simulink model "SCRReferenceApplication"  (R2021a)
settings: Solver=ode23tb  StartTime=0.0  StopTime=20  RelTol=2e-1
model workspace (MAT data in the model file):
  EngPwr = 352122.842504
  EngWc = 4.047
  Tdiff = 849
  Tlim = 1000
  VEH.Mass = 1181
  VEH.StaticNormalFrontLoad.FR = 264.666666667
  VEH.StaticNormalFrontLoad.FL = 264.666666667
  VEH.StaticNormalRearLoad.RR = 322
  VEH.StaticNormalRearLoad.RL = 322
  VEH.WheelBase = 3.075
  VEH.FrontAxlePositionfromCG = 1.515
  VEH.RearAxlePositionfromCG = 1.504
  VEH.HeightCG = 0.134
  VEH.FrontalArea = 2.11
  VEH.DragCoefficient = 0.33
  VEH.NumberOfWheelsPerAxle = 2
  VEH.Thread.FR = 1.705
  VEH.Thread.RR = 1.705
  VEH.PitchMomentInertia = 1922.66666667
  VEH.RollMomentInertia = 432.333333333
  VEH.YawMomentInertia = 2066
  VEH.SteeringRatio = 18
  VEH.TrackWidth = 1.922
  VEH.SprungMass = 1096.72266667
  VEH.InitialLongPosition = 0
  VEH.InitialLatPosition = 3.125
  VEH.InitialVertPosition = 0.0111
  VEH.InitialRollAngle = 0
  VEH.InitialPitchAngle = -0.000732
  VEH.InitialYawAngle = 0
  VEH.InitialLongVel = 0
  VEH.InitialLatVel = 0
  VEH.InitialVertVel = 0
  VEH.InitialRollRate = 0
  VEH.InitialPitchRate = 0
  VEH.InitialYawRate = 0
libraries: sim3dlib x3, Solver_SF x1, vdynlib x1, simulink x1
settings Model: ModifiedByFormat=The MathWorks, Inc.  SimulationMode=accelerator  Creator=The MathWorks, Inc.  LastModifiedBy=The MathWorks, Inc.
settings SolverCC: SolverJacobianMethodControl=FullPerturbation  ZeroCrossAlgorithm=Adaptive  AlgebraicLoopSolver=TrustRegion  DecoupledContinuousIntegration=on  MinimalZcImpactIntegration=on
settings DataIOCC: ReturnWorkspaceOutputs=off  Refine=2
settings DebuggingCC: IgnoredZcDiagnostic=none  PregeneratedLibrarySubsystemCodeDiagnostic=none  SFMachineParentedDataDiag=warning  ArithmeticOperatorsInVariantConditions=warning
settings ModelReferenceCC: ModelReferenceMinAlgLoopOccurrences=on
settings SFSimCC: SimUseLocalCustomCode=off
settings RTWCC: RTWUseLocalCustomCode=off

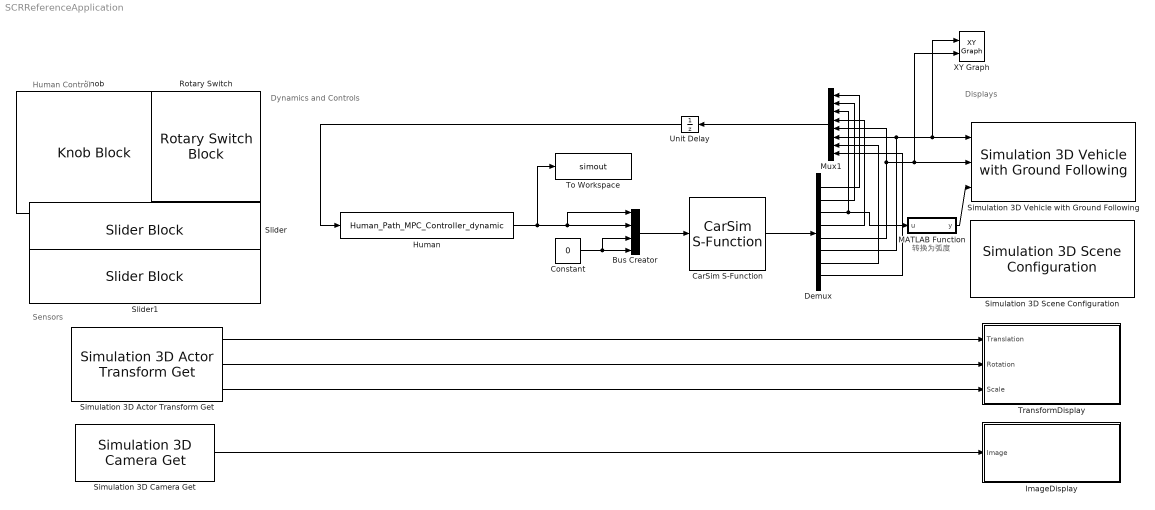
== system SCRReferenceApplication ==
  note: 转换为弧度
  note: Displays
  note: Dynamics and Controls
  note: Sensors
  note: Human Control
  Bus Creator : BusCreator  Inputs=4
  CarSim S-Function : Solver_SF/CarSim S-Function  Priority=1  SIMFILE=simfile.sim  Run_RTs=off  vs_state_ind=Run  StopMode_ind=Vehicle Model
  Constant : Constant  Value=0
  Demux : Demux  Outputs=8
  Human : S-Function  FunctionName=Human_Path_MPC_Controller_dynamic  SFunctionDeploymentMode=off  EnableBusSupport=off
  ImageDisplay : Subsystem
  Knob : KnobBlock  LabelPosition=Bottom  ScaleMin=-90  ScaleMax=90  TickInterval=30
  MATLAB Function : MATLAB Function  TreatAsAtomicUnit=on
  Mux1 : Mux  Inputs=8
  Rotary Switch : RotarySwitchBlock  LabelPosition=Bottom
      settings: Values={{'R', 'N', 'D'}, [-1 0 1]}
  Simulation 3D Actor Transform Get : sim3dlib/Simulation 3D Actor Transform Get  Priority=1  ActorTag=SimulinkVehicle1  NumberOfParts=5  CustNumOfParts=3  Ts=-1  aMode=2
      settings: SourceProductBaseCode=DR,UV,VE
  Simulation 3D Camera Get : sim3dlib/Simulation 3D Camera Get  Priority=1  sensorTag=Sim3dSensor1  sensorId=1  sensorName=Sim3dSensor1  vehTagList={'Scene Origin';'SimulinkVehicle1'}  vehTag=SimulinkVehicle1  mountLoc=Rearview mirror  offsetFlag=off  tmountOffset=[0, 0, 0]  rmountOffset=[0, 0, 0]  HorizontalResolution=1024  VerticalResolution=768  HorizontalFOV=90  SampleTime=.03  mountPoint=[0.319999992847443 0 1.19000005722046]  mountOrientation=[0 0 0]  aMode=2  ID=1
      settings: SourceProductBaseCode=DR,UV,VE
  Simulation 3D Scene Configuration : sim3dlib/Simulation 3D Scene Configuration  Priority=0  ProjectFormat=Default Scenes  SceneDesc=Straight road  ProjectName=F:\MATLAB\R2021a\toolbox\shared\sim3d_projects\automotive_project\UE4\WindowsNoEditor\VehicleSimulation.exe  ScenePath=/Game/Maps/HwStrght  vehTagList={'Scene Origin';'SimulinkVehicle1'}  vehTag=SimulinkVehicle1  OpVisEn=off  Ts=.03  EnableWindow=on  EnableWeather=off  SunAltitude=60  SunAzimuth=90  clouds=40  wind=1  fog=0  rain=0  sensorTag=MainCamera1  sensorId=1  sensorName=MainCamera1  mountLoc=Origin  offsetFlag=off  tmountOffset=[0, 0, 0]  rmountOffset=[0, 0, 0]  HorizontalResolution=1280  VerticalResolution=720  HorizontalFOV=60  mountPoint=[0 0 0]  mountOrientation=[0 0 0]  aMode=2  ID=1
      settings: SourceProductBaseCode=DR,UV,VE
  Simulation 3D Vehicle with Ground Following : vdynlib/Vehicle Scenarios/Sim3D/Sim3D Vehicle/Components/Simulation 3D Vehicle with Ground Following  Priority=-1  PassVehMesh=Muscle car  MeshPath=/MathWorksSimulation/Vehicles/Muscle/Meshes/SK_MuscleCar.SK_MuscleCar  TrackWidth=1.9  WheelBase=3  WheelRadius=0.35  VehColor=Red  InitialPos=[0, 0, 0]  InitialRot=[0, 0, 0]  ActorName=SimulinkVehicle1  VehLightsControl=off  HeadlightColor=[ 1, 1, 1 ]  HighBeamIntensity=100000  LowBeamIntensity=60000  HighBeamConeAngle=1.22  LowBeamConeAngle=1.22  LeftHeadlightOrientation=[ 0, 0 ]  RightHeadlightOrientation=[ 0, 0 ]  BrakelightIntensity=200  ReverselightIntensity=500  SignallightIntensity=500  SignallightPeriod=1  SignalPulseWidth=50  SampleTime=-1  ActorType=SimulinkVehicle  ID=1  aMode=2  ActorTag=SimulinkVehicle1  CoordinateScheme=SAE
      settings: SourceProductBaseCode=VE
  Slider : SliderBlock  LabelPosition=Bottom  ScaleMax=1  TickInterval=.2
  Slider1 : SliderBlock  LabelPosition=Bottom  ScaleMax=1  TickInterval=.2
  To Workspace : ToWorkspace  VariableName=simout  SaveFormat=Timeseries  SampleTime=-1
  TransformDisplay : Subsystem
  Unit Delay : UnitDelay  SampleTime=-1  HasFrameUpgradeWarning=on
  XY Graph : simulink/Sinks/XY Graph  xmin=-5  xmax=200  ymin=-2  ymax=10  st=-1
  wires:
  Simulation 3D Camera Get/1 -> ImageDisplay/1(Image)
  Simulation 3D Actor Transform Get/1 -> TransformDisplay/1(Translation)
  Simulation 3D Actor Transform Get/2 -> TransformDisplay/2(Rotation)
  Simulation 3D Actor Transform Get/3 -> TransformDisplay/3(Scale)
  CarSim S-Function/1 -> Demux/1
  Mux1/1 -> Unit Delay/1
  Unit Delay/1 -> Human/1
  MATLAB Function/1(y) -> Simulation 3D Vehicle with Ground Following/3
  Demux/2 -> Mux1/2
  Demux/3 -> MATLAB Function/1(u), Mux1/3
  Demux/4 -> Mux1/4
  Demux/5 -> XY Graph/2, Simulation 3D Vehicle with Ground Following/2, Mux1/5
  Demux/6 -> XY Graph/1, Simulation 3D Vehicle with Ground Following/1, Mux1/6
  Demux/1 -> Mux1/1
  Demux/7 -> Mux1/7
  Demux/8 -> Mux1/8
  Constant/1 -> Bus Creator/3, Bus Creator/4
  Bus Creator/1 -> CarSim S-Function/1
  Human/1 -> To Workspace/1, Bus Creator/1, Bus Creator/2

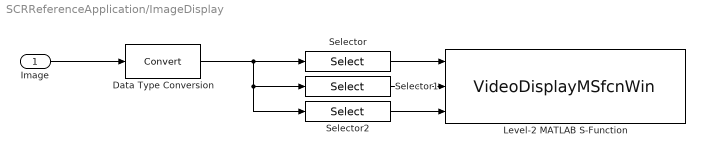
== system SCRReferenceApplication/ImageDisplay ==
  Image : Inport
  Data Type Conversion : DataTypeConversion
  Level-2 MATLAB S-Function : M-S-Function  FunctionName=VideoDisplayMSfcnWin  Parameters=1
  Selector : Selector  NumberOfDimensions=3  InputPortWidth=3  IndexOptions=Select all,Select all,Index vector (dialog)  Indices=[1 3],1,1  OutputSizes=1,1,1
  Selector1 : Selector  NumberOfDimensions=3  InputPortWidth=3  IndexOptions=Select all,Select all,Index vector (dialog)  Indices=[1 3],1,2  OutputSizes=1,1,1
  Selector2 : Selector  NumberOfDimensions=3  InputPortWidth=3  IndexOptions=Select all,Select all,Index vector (dialog)  Indices=[1 3],1,3  OutputSizes=1,1,1
  wires:
  Data Type Conversion/1 -> Selector2/1, Selector1/1, Selector/1
  Image/1 -> Data Type Conversion/1
  Selector1/1 -> Level-2 MATLAB S-Function/2
  Selector2/1 -> Level-2 MATLAB S-Function/3
  Selector/1 -> Level-2 MATLAB S-Function/1

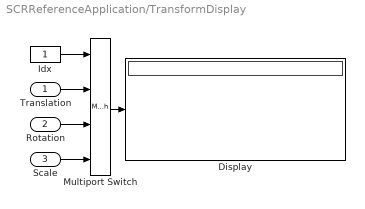
== system SCRReferenceApplication/TransformDisplay ==
  Translation : Inport
  Rotation : Inport  Port=2
  Scale : Inport  Port=3
  " Multiport Switch" : MultiPortSwitch
  Display : Display
  Idx : Constant
  wires:
  " Multiport Switch"/1 -> Display/1
  Idx/1 -> " Multiport Switch"/1
  Scale/1 -> " Multiport Switch"/4
  Translation/1 -> " Multiport Switch"/2
  Rotation/1 -> " Multiport Switch"/3

== matlab function SCRReferenceApplication/MATLAB Function ==
  data: u input; y output
function y = fcn(u)

y = u/180*pi;
